simulink model "temp"  (R2020b)
settings: Solver=VariableStepAuto  StartTime=0.0  StopTime=inf  RelTol=1e-3
libraries: simulink x2, TcSimInterface x1
(part 2 of 2)

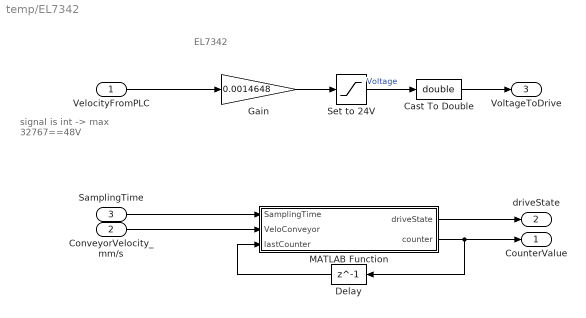
== system temp/EL7342 ==
  note: signal is int ->
      | max 32767==48V
  note: EL7342
  VelocityFromPLC : Inport
  ConveyorVelocity_mm/s : Inport  Port=2
  SamplingTime : Inport  Port=3
  Cast To Double : DataTypeConversion  OutDataTypeStr=double
  Delay : Delay  DelayLength=1
  Gain : Gain  Gain=0.0014648
  MATLAB Function : MATLAB Function  TreatAsAtomicUnit=on
  Set to 24V : Saturate  UpperLimit=24  LowerLimit=-24
  CounterValue : Outport
  driveState : Outport  Port=2
  VoltageToDrive : Outport  Port=3
  wires:
  Gain/1 -> Set to 24V/1
  Cast To Double/1 -> VoltageToDrive/1
  MATLAB Function/2(counter) -> Delay/1, CounterValue/1
  ConveyorVelocity_mm/s/1 -> MATLAB Function/2(VeloConveyor)
  MATLAB Function/1(driveState) -> driveState/1
  Set to 24V/1 -> Cast To Double/1  "Voltage"
  Delay/1 -> MATLAB Function/3(lastCounter)
  SamplingTime/1 -> MATLAB Function/1(SamplingTime)
  VelocityFromPLC/1 -> Gain/1

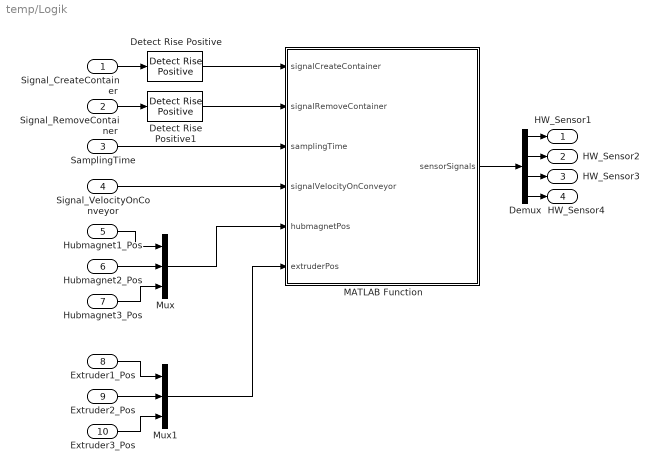
== system temp/Logik ==
  Signal_CreateContainer : Inport
  Signal_RemoveContainer : Inport  Port=2
  SamplingTime : Inport  Port=3
  Signal_VelocityOnConveyor : Inport  Port=4
  Hubmagnet1_Pos : Inport  Port=5
  Hubmagnet2_Pos : Inport  Port=6
  Hubmagnet3_Pos : Inport  Port=7
  Extruder1_Pos : Inport  Port=8
  Extruder2_Pos : Inport  Port=9
  Extruder3_Pos : Inport  Port=10
  Demux : Demux
  Detect Rise Positive : simulink/Logic and Bit Operations/Detect Rise Positive  vinit=0  OutDataTypeStr=boolean
  Detect Rise Positive1 : simulink/Logic and Bit Operations/Detect Rise Positive  vinit=0  OutDataTypeStr=boolean
  MATLAB Function : MATLAB Function  TreatAsAtomicUnit=on
  Mux : Mux  Inputs=3
  Mux1 : Mux  Inputs=3
  HW_Sensor1 : Outport
  HW_Sensor2 : Outport  Port=2
  HW_Sensor3 : Outport  Port=3
  HW_Sensor4 : Outport  Port=4
  wires:
  Demux/4 -> HW_Sensor4/1
  Detect Rise Positive1/1 -> MATLAB Function/2(signalRemoveContainer)
  Detect Rise Positive/1 -> MATLAB Function/1(signalCreateContainer)
  Demux/3 -> HW_Sensor3/1
  Demux/2 -> HW_Sensor2/1
  Demux/1 -> HW_Sensor1/1
  MATLAB Function/1(sensorSignals) -> Demux/1
  Mux1/1 -> MATLAB Function/6(extruderPos)
  Mux/1 -> MATLAB Function/5(hubmagnetPos)
  Signal_VelocityOnConveyor/1 -> MATLAB Function/4(signalVelocityOnConveyor)
  SamplingTime/1 -> MATLAB Function/3(samplingTime)
  Signal_RemoveContainer/1 -> Detect Rise Positive1/1
  Signal_CreateContainer/1 -> Detect Rise Positive/1
  Extruder3_Pos/1 -> Mux1/3
  Extruder1_Pos/1 -> Mux1/1
  Extruder2_Pos/1 -> Mux1/2
  Hubmagnet3_Pos/1 -> Mux/3
  Hubmagnet2_Pos/1 -> Mux/2
  Hubmagnet1_Pos/1 -> Mux/1

== matlab function temp/EL7342/MATLAB Function ==
  data: driveState output; SamplingTime input; VeloConveyor input; counter output; lastCounter input
function [driveState,counter] = fcn(SamplingTime, VeloConveyor, lastCounter)
%%
%    VeloConveyor in mm/s
%    SamplingTime in s
%    lastCounter 1count = 0.0001mm

%%
driveState = uint8(0);
driveState = bitset(driveState,1,1);    % Ready to enable
driveState = bitset(driveState,2,1);    % Ready 
if (VeloConveyor > 0)
    driveState = bitset(driveState,5,1);    % Moving Positive
elseif (VeloConveyor < 0)
    driveState = bitset(driveState,6,1);    % Moving Negative
end

diff = VeloConveyor*SamplingTime*10000;
if (lastCounter+diff >= 65535)
    counter = lastCounter+diff -65535;
else
    counter = lastCounter + VeloConveyor*SamplingTime*10000;
end

end

== matlab function temp/Encode ==
  data: counterValue input; modelToPlc output; driveState input
function modelToPlc = EncodePlcMessage(counterValue, driveState)
    modelToPlc = uint32(0);
    modelToPlc = bitor(modelToPlc, uint32(driveState));
    modelToPlc = bitshift(modelToPlc,16);
    
    modelToPlc = bitor(modelToPlc, uint32(counterValue));
    
    %modelToPlc = bitand(modelToPlc, bitshift(driveState,16));
    %modelToPlc = bitand(modelToPlc, counterValue);

end

== matlab function temp/Decode ==
  data: PlcToModel input; velocity output
function velocity  = DecodePlcMessage(PlcToModel)


velocity = bitand(PlcToModel, uint32(0xffff));

end

== matlab function temp/Logik/MATLAB Function ==
  settings: updateMethod=DISCRETE
  data: signalCreateContainer input; sensorSignals output; signalRemoveContainer input; samplingTime input; signalVelocityOnConveyor input; hubmagnetPos input; extruderPos input
function sensorSignals = fcn(signalCreateContainer, signalRemoveContainer, samplingTime, signalVelocityOnConveyor, hubmagnetPos, extruderPos)
    % samplingTime in s
    % signalVelocityOnConveyor in mm/s
    % hubmagnetPos between 1 () and 0 ()
    
    %% Mechanical Properties
    posStopperOnConveyor = [100 200 300 400]';
    
    %%  Variables
    persistent containers                   % Store Position in mm
    persistent containersValid
    sensorSignals = [false, false, false, false]';
    stopperStatePassable = [hubmagnetPos; 0];       % 0=Stopping
    
    if (isempty(containersValid))
        containersValid = false;
    end
    
    if (isempty(containers))
        containers = [0];
    end
    
    %% Create Container on Signal
    if (signalCreateContainer == true)
        if (containersValid == false)
            containersValid = true;
        else
            containers = [containers 0];
        end
    end
    
    %% Remove Container On Signal
    if (signalRemoveContainer==true)
        if (max(size(containers)) > 1)
            containers(1) = [];
        else
            containersValid = false;
        end
    end
    
    %% Logic
    if (containersValid == true)
        for idxContainer = 1:max(size(containers))
            containerPos = containers(idxContainer);
            travelDistance = signalVelocityOnConveyor*samplingTime;
            
            for idxStopper = 1:max(size(posStopperOnConveyor))
                if (containerPos < posStopperOnConveyor(idxStopper))
                    distanceToStopper = posStopperOnConveyor(idxStopper)-containerPos;
                    
                    % Stop before stopper
                    if (stopperStatePassable(idxStopper) == false && travelDistance >= distanceToStopper)
                        travelDistance = 0;
                    end                    
                    
                    % Set Sensor if needed
                    if (distanceToStopper < 3)                    
                        sensorSignals(idxStopper) = true;
                    end
                    
                    break;
                end                    
            end    
            
            % Change position of container if possible
            containers(idxContainer) = containers(idxContainer) + travelDistance;
        end        
    end
end
